simulink model "bit_mapping_demo"  (R2025b)
settings: Solver=VariableStepAuto  StartTime=0.0  StopTime=10.0  RelTol=1e-3
settings Model: Creator=cherrywj  LastModifiedBy=cherrywj

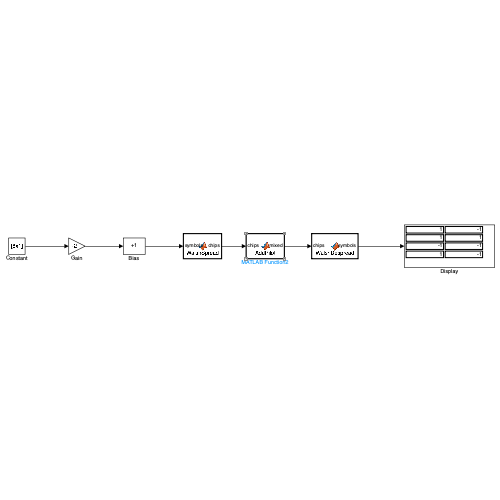
[thumbnail: Simulink's stored preview of the top-level diagram]
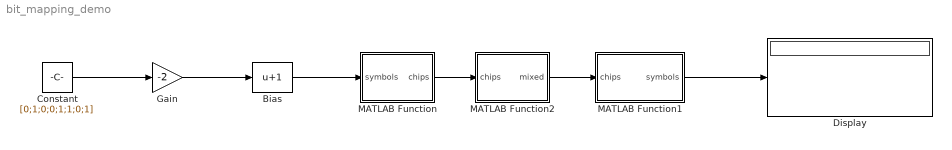
== system bit_mapping_demo ==
  Bias : Bias  Bias=1  SaturateOnIntegerOverflow=off
  Constant : Constant  Value=[0;1;0;0;1;1;0;1]  VectorParams1D=off
  Display : Display
  Gain : Gain  Gain=-2
  MATLAB Function : MATLAB Function  TreatAsAtomicUnit=on
  MATLAB Function1 : MATLAB Function  TreatAsAtomicUnit=on
  MATLAB Function2 : MATLAB Function  TreatAsAtomicUnit=on
  wires:
  Constant/1 -> Gain/1
  Gain/1 -> Bias/1
  Bias/1 -> MATLAB Function/1(symbols)
  MATLAB Function1/1(symbols) -> Display/1
  MATLAB Function/1(chips) -> MATLAB Function2/1(chips)
  MATLAB Function2/1(mixed) -> MATLAB Function1/1(chips)

== matlab function bit_mapping_demo/MATLAB Function ==
  data: symbols input; chips output
function chips = WalshSpread(symbols)
% Spread eight symbols with a length-64 Walsh sequence.

w = repmat([1; -1], 32, 1);
chips = zeros(512, 1);

for k = 1:8
    idx = (k - 1) * 64 + (1:64);
    chips(idx) = symbols(k) * w;
end
end

== matlab function bit_mapping_demo/MATLAB Function2 ==
  data: chips input; mixed output
function mixed = AddPilot(chips)
% Add an all-ones pilot branch in the Walsh domain.

pilotAmplitude = 0.5;
pilot = ones(512, 1);

mixed = chips + pilotAmplitude * pilot;
end

== matlab function bit_mapping_demo/MATLAB Function1 ==
  data: chips input; symbols output
function symbols = WalshDespread(chips)
% Recover eight symbols by correlation.

w = repmat([1; -1], 32, 1);
symbols = zeros(8, 1);

for k = 1:8
    acc = 0;
    for m = 1:64
        idx = (k - 1) * 64 + m;
        acc = acc + chips(idx) * w(m);
    end
    symbols(k) = acc / 64;
end
end
